simulink model "RoboProgram1"  (R2020b)
settings: Solver=FixedStepAuto  StartTime=0.0  StopTime=inf  RelTol=1e-3  EnableMultiTasking=on
libraries: vexarmcortexlib x16, vexcommonlib x3
settings Model: Creator=joshm  LastModifiedBy=joshm
settings DataIOCC: LimitDataPoints=on  SignalLoggingSaveFormat=ModelDataLogs  ReturnWorkspaceOutputs=off
settings OptimizationCC: ExpressionDepthLimit=2147483647  LifeSpan=Inf  MaxStackSize=64  EfficientTunableParamExpr=on
settings DebuggingCC: UnderspecifiedInitializationDetection=Classic  MergeDetectMultiDrivingBlocksExec=none  InheritedTsInSrcMsg=none  FcnCallInpInsideContextMsg=warning  UnconnectedInputMsg=none  UnconnectedOutputMsg=none  StateNameClashWarn=warning  SFUnexpectedBacktrackingDiag=warning  SFNoUnconditionalDefaultTransitionDiag=warning  SFExecutionAtInitializationDiag=none  ArithmeticOperatorsInVariantConditions=warning
settings HardwareCC: ProdBitPerPointer=32  ProdBitPerSizeT=32  ProdBitPerPtrDiffT=32  ProdLargestAtomicInteger=Long  ProdLargestAtomicFloat=Double  ProdIntDivRoundTo=Undefined  ProdWordSize=32  ProdHWDeviceType=ARM Compatible->ARM Cortex
settings ModelReferenceCC: PropagateSignalLabelsOutOfModel=off
settings SFSimCC: MATLABDynamicMemAlloc=off  CustomCodeUndefinedFunction=UseInterfaceOnly
settings RTWCC: Description=Embedded Coder  SystemTargetFile=ert.tlc  HardwareBoard=ARM Cortex-based VEX Microcontroller  TemplateMakefile=ert_default_tmf  Toolchain=GNU Tools for VEX ARM Cortex
settings CodeAppCC: IgnoreCustomStorageClasses=off  CustomSymbolStrType=$N$R$M  StateflowObjectComments=on  InternalIdentifier=Classic
settings ERTTargetCC: CodeReplacementLibrary=GCC ARM Cortex-M3  MultiwordLength=2048  ConvertIfToSwitch=off  SuppressUnreachableDefaultCases=off

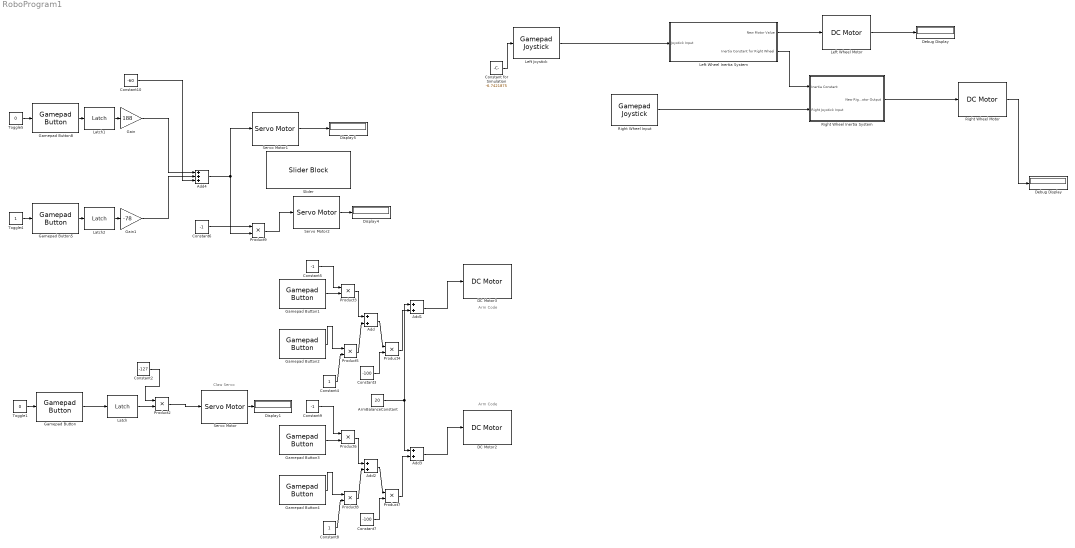
== system RoboProgram1 ==
  note: Claw Servo
  note: Arm Code
  note: Arm Code
  " Debug Display" : Display
  Add{,1..3} (4 alike) : Sum
  Add4 : Sum  Inputs=+++
  ArmBalanceConstant : Constant  Value=20
  Constant for Simulation : Constant  Value=-6.7421875  SampleTime=0.02
  Constant10 : Constant  Value=-60
  Constant2 : Constant  Value=-127
  Constant3 : Constant  Value=-100
  Constant4 : Constant
  Constant5 : Constant  Value=-1
  Constant6 : Constant  Value=-1
  Constant7 : Constant  Value=-100
  Constant8 : Constant
  Constant9 : Constant  Value=-1
  DC Motor2 : vexarmcortexlib/Actuators/DC Motor  motor=6  scaleFactor=1/13.5  SimulationOut=on
      settings: SourceProductBaseCode=EC_VEX_MICRO
  DC Motor3 : vexarmcortexlib/Actuators/DC Motor  motor=4  scaleFactor=1/13.5  SimulationOut=on
      settings: SourceProductBaseCode=EC_VEX_MICRO
  Debug Display : Display
  Display1 : Display
  Display4 : Display
  Display5 : Display
  Gain : Gain  Gain=188
  Gain1 : Gain  Gain=-78
  Gamepad Button : vexarmcortexlib/Gamepad/Gamepad Button  joystick=1  chan=6  button56=Up  button78=Down  SimulationIn=on  SampleTime=0.02
      settings: SourceProductBaseCode=EC_VEX_MICRO
  Gamepad Button1 : vexarmcortexlib/Gamepad/Gamepad Button  joystick=1  chan=5  button56=Up  button78=Down  SimulationIn=off  SampleTime=0.02
      settings: SourceProductBaseCode=EC_VEX_MICRO
  Gamepad Button2 : vexarmcortexlib/Gamepad/Gamepad Button  joystick=1  chan=5  button56=Down  button78=Down  SimulationIn=off  SampleTime=0.02
      settings: SourceProductBaseCode=EC_VEX_MICRO
  Gamepad Button3 : vexarmcortexlib/Gamepad/Gamepad Button  joystick=1  chan=5  button56=Up  button78=Down  SimulationIn=off  SampleTime=0.02
      settings: SourceProductBaseCode=EC_VEX_MICRO
  Gamepad Button4 : vexarmcortexlib/Gamepad/Gamepad Button  joystick=1  chan=5  button56=Down  button78=Down  SimulationIn=off  SampleTime=0.02
      settings: SourceProductBaseCode=EC_VEX_MICRO
  Gamepad Button5 : vexarmcortexlib/Gamepad/Gamepad Button  joystick=1  chan=8  button56=Up  button78=Up  SimulationIn=on  SampleTime=0.02
      settings: SourceProductBaseCode=EC_VEX_MICRO
  Gamepad Button8 : vexarmcortexlib/Gamepad/Gamepad Button  joystick=1  chan=8  button56=Up  button78=Down  SimulationIn=on  SampleTime=0.02
      settings: SourceProductBaseCode=EC_VEX_MICRO
  Latch : vexcommonlib/Latch  output0=off  BlockPlatform=vexarmcortex
      settings: SourceProductBaseCode=EC_VEX_MICRO,VEXV5
  Latch1 : vexcommonlib/Latch  output0=off  BlockPlatform=vexarmcortex
      settings: SourceProductBaseCode=EC_VEX_MICRO,VEXV5
  Latch2 : vexcommonlib/Latch  output0=off  BlockPlatform=vexarmcortex
      settings: SourceProductBaseCode=EC_VEX_MICRO,VEXV5
  Left Joystick : vexarmcortexlib/Gamepad/Gamepad Joystick  joystick=1  chan=3  SimulationIn=on  SampleTime=0.02
      settings: SourceProductBaseCode=EC_VEX_MICRO
  Left Wheel Inertia System : Subsystem
  Left Wheel Motor : vexarmcortexlib/Actuators/DC Motor  motor=2  scaleFactor=1/13.5  SimulationOut=on
      settings: SourceProductBaseCode=EC_VEX_MICRO
  Product{2..9} (8 alike) : Product  RndMeth=Zero
  Right Wheel Inertia System : Subsystem
  Right Wheel Input : vexarmcortexlib/Gamepad/Gamepad Joystick  joystick=1  chan=2  SimulationIn=off  SampleTime=0.02
      settings: SourceProductBaseCode=EC_VEX_MICRO
  Right Wheel Motor : vexarmcortexlib/Actuators/DC Motor  motor=3  scaleFactor=1/13.5  SimulationOut=on
      settings: SourceProductBaseCode=EC_VEX_MICRO
  Servo Motor : vexarmcortexlib/Actuators/Servo Motor  motor=5  scaleFactor=60/127  SimulationOut=on
      settings: SourceProductBaseCode=EC_VEX_MICRO
  Servo Motor1 : vexarmcortexlib/Actuators/Servo Motor  motor=7  scaleFactor=60/127  SimulationOut=on
      settings: SourceProductBaseCode=EC_VEX_MICRO
  Servo Motor2 : vexarmcortexlib/Actuators/Servo Motor  motor=8  scaleFactor=60/127  SimulationOut=on
      settings: SourceProductBaseCode=EC_VEX_MICRO
  Slider : SliderBlock  ScaleMin=-128  ScaleMax=127
  Toggle1 : Constant  Value=0
      settings: OpenFcn=|
      | if strcmp('0',get_param(gcb, 'Value'))                        set_param(gcb, 'Value', '1');
      | else
      |             set_param(gcb, 'Value', '0');
      | end
  Toggle4 : Constant
      settings: OpenFcn=|
      | if strcmp('0',get_param(gcb, 'Value'))                        set_param(gcb, 'Value', '1');
      | else
      |             set_param(gcb, 'Value', '0');
      | end
  Toggle5 : Constant  Value=0
      settings: OpenFcn=|
      | if strcmp('0',get_param(gcb, 'Value'))                        set_param(gcb, 'Value', '1');
      | else
      |             set_param(gcb, 'Value', '0');
      | end
  wires:
  Gamepad Button/1 -> Latch/1
  Constant2/1 -> Product2/1
  Product2/1 -> Servo Motor/1
  Constant3/1 -> Product4/2
  Gamepad Button2/1 -> Product5/1
  Product4/1 -> Add1/2
  Gamepad Button1/1 -> Product3/2
  Latch/1 -> Product2/2
  Product5/1 -> Add/2
  Product3/1 -> Add/1
  Constant5/1 -> Product3/1
  Constant4/1 -> Product5/2
  Add/1 -> Product4/1
  Add1/1 -> DC Motor3/1
  ArmBalanceConstant/1 -> Add1/1, Add3/1
  Add3/1 -> DC Motor2/1
  Constant9/1 -> Product6/1
  Product6/1 -> Add2/1
  Constant7/1 -> Product7/2
  Constant8/1 -> Product8/2
  Gamepad Button4/1 -> Product8/1
  Product8/1 -> Add2/2
  Product7/1 -> Add3/2
  Gamepad Button3/1 -> Product6/2
  Add2/1 -> Product7/1
  Toggle1/1 -> Gamepad Button/1
  Servo Motor/1 -> Display1/1
  Toggle5/1 -> Gamepad Button8/1
  Toggle4/1 -> Gamepad Button5/1
  Gamepad Button5/1 -> Latch2/1
  Gamepad Button8/1 -> Latch1/1
  Gain/1 -> Add4/1
  Gain1/1 -> Add4/2
  Product9/1 -> Servo Motor2/1
  Constant6/1 -> Product9/1
  Add4/1 -> Servo Motor1/1, Product9/2
  Servo Motor2/1 -> Display4/1
  Servo Motor1/1 -> Display5/1
  Latch1/1 -> Gain/1
  Latch2/1 -> Gain1/1
  Constant10/1 -> Add4/3
  Constant for Simulation/1 -> Left Joystick/1
  Right Wheel Motor/1 -> Debug Display/1
  Right Wheel Input/1 -> Right Wheel Inertia System/2(Right Joystick Input)
  Right Wheel Inertia System/1(New Right Motor Output) -> Right Wheel Motor/1
  Left Wheel Inertia System/1(New Motor Value) -> Left Wheel Motor/1
  Left Joystick/1 -> Left Wheel Inertia System/1(Joystick Input)
  Left Wheel Motor/1 -> " Debug Display"/1
  Left Wheel Inertia System/2(Inertia Constant for Right Wheel) -> Right Wheel Inertia System/1(Inertia Constant)

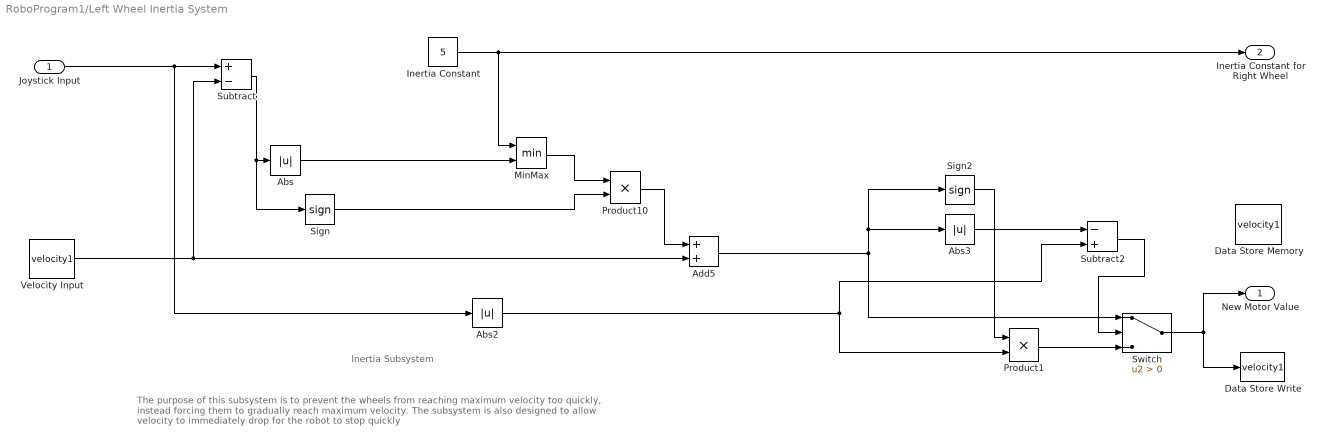
== system RoboProgram1/Left Wheel Inertia System ==
  note: The purpose of this subsystem is to prevent the wheels from reaching maximum velocity too quickly, instead forcing them to gradually reach maximum velocity. The subsystem is also designed to allow velocity to immediately drop for the robot to stop quickly
  note: Inertia Subsystem
  Joystick Input : Inport
  Abs : Abs
  Abs2 : Abs
  Abs3 : Abs
  Add5 : Sum
  Data Store Memory : DataStoreMemory  DataStoreName=velocity1  ReadBeforeWriteMsg=warning  WriteAfterWriteMsg=warning  WriteAfterReadMsg=warning  ShowAdditionalParam=off
  Data Store Write : DataStoreWrite  DataStoreName=velocity1  SampleTime=0.02
  Inertia Constant : Constant  Value=5
  MinMax : MinMax  Inputs=2
  Product1 : Product  RndMeth=Zero
  Product10 : Product  RndMeth=Zero
  Sign : Signum
  Sign2 : Signum
  Subtract : Sum  Inputs=+-
  Subtract2 : Sum  Inputs=-+
  Switch : Switch  Criteria=u2 > Threshold
  Velocity Input : DataStoreRead  DataStoreName=velocity1  SampleTime=0.02
  New Motor Value : Outport
  Inertia Constant for Right Wheel : Outport  Port=2
  wires:
  Joystick Input/1 -> Abs2/1, Subtract/1
  Subtract/1 -> Sign/1, Abs/1
  Add5/1 -> Abs3/1, Sign2/1, Switch/1
  Abs/1 -> MinMax/2
  Sign/1 -> Product10/2
  Velocity Input/1 -> Subtract/2, Add5/2
  Abs2/1 -> Subtract2/2, Product1/2
  Product10/1 -> Add5/1
  Sign2/1 -> Product1/1
  MinMax/1 -> Product10/1
  Inertia Constant/1 -> MinMax/1, Inertia Constant for Right Wheel/1
  Switch/1 -> New Motor Value/1, Data Store Write/1
  Subtract2/1 -> Switch/2
  Abs3/1 -> Subtract2/1
  Product1/1 -> Switch/3

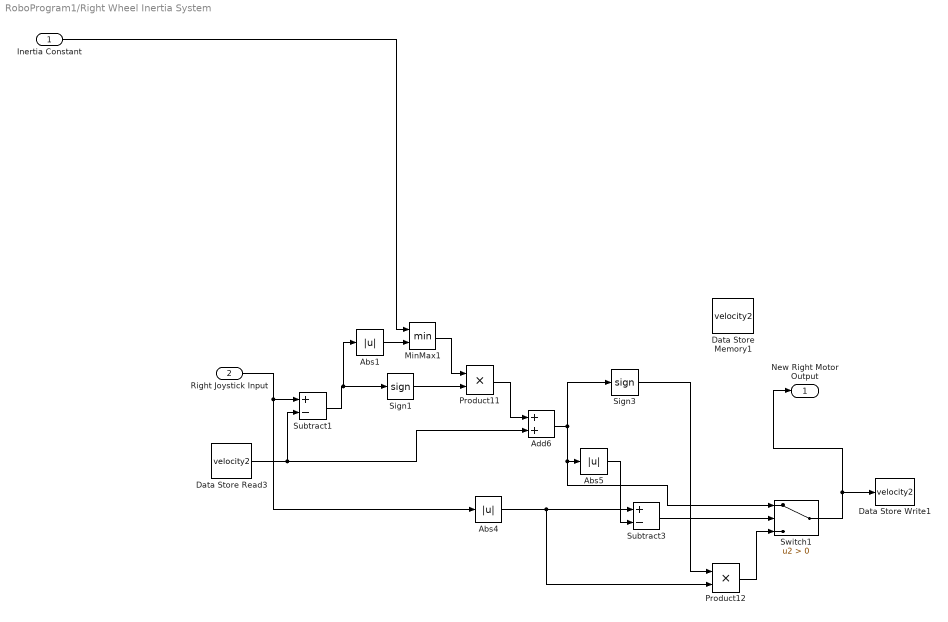
== system RoboProgram1/Right Wheel Inertia System ==
  Inertia Constant : Inport
  Right Joystick Input : Inport  Port=2
  Abs1 : Abs
  Abs4 : Abs
  Abs5 : Abs
  Add6 : Sum
  Data Store Memory1 : DataStoreMemory  DataStoreName=velocity2  ReadBeforeWriteMsg=warning  WriteAfterWriteMsg=warning  WriteAfterReadMsg=warning  ShowAdditionalParam=off
  Data Store Read3 : DataStoreRead  DataStoreName=velocity2  SampleTime=0.02
  Data Store Write1 : DataStoreWrite  DataStoreName=velocity2  SampleTime=0.02
  MinMax1 : MinMax  Inputs=2
  Product11 : Product  RndMeth=Zero
  Product12 : Product  RndMeth=Zero
  Sign1 : Signum
  Sign3 : Signum
  Subtract1 : Sum  Inputs=+-
  Subtract3 : Sum  Inputs=+-
  Switch1 : Switch  Criteria=u2 > Threshold
  New Right Motor Output : Outport
  wires:
  MinMax1/1 -> Product11/1
  Abs5/1 -> Subtract3/2
  Product11/1 -> Add6/1
  Abs4/1 -> Product12/2, Subtract3/1
  Abs1/1 -> MinMax1/2
  Subtract3/1 -> Switch1/2
  Subtract1/1 -> Abs1/1, Sign1/1
  Sign1/1 -> Product11/2
  Sign3/1 -> Product12/1
  Data Store Read3/1 -> Subtract1/2, Add6/2
  Add6/1 -> Abs5/1, Switch1/1, Sign3/1
  Right Joystick Input/1 -> Abs4/1, Subtract1/1
  Inertia Constant/1 -> MinMax1/1
  Product12/1 -> Switch1/3
  Switch1/1 -> New Right Motor Output/1, Data Store Write1/1
